simulink subsystem "Battery4Cell_SW_Res"  (R2022b)
settings: Solver=VariableStepAuto  StartTime=0.0  StopTime=10.0  RelTol=1e-3
model mask{V0=3.7, Ah=5.20, SOC1=70, SOC2=50, SOC3=60, SOC4=85, R=1}
  mask prompts: V0 "Nominal Voltage (V)"; Ah "Rated Capacity (Ah)"; SOC1 "Init SOC1 (%)"; SOC2 "Init SOC2 (%)"; SOC3 "Init SOC3 (%)"; SOC4 "Init SOC4 (%)"; R "Shunting Resistance"
undefined symbols (not defined in the file): Ion, Lithium
libraries: spsBatteryLib x4, spsIdealSwitchLib x4, spsParallelRLCBranchLib x4
settings Model: Creator=MAAM  LastModifiedBy=MAAM

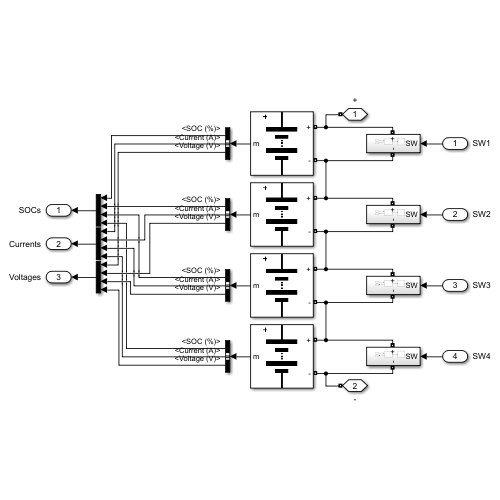
[thumbnail: Simulink's stored preview of the top-level diagram]
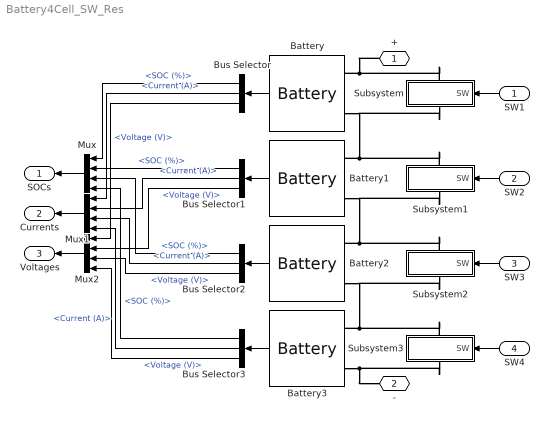
== system Battery4Cell_SW_Res ==
  SW1 : Inport
  SW2 : Inport  Port=2
  SW3 : Inport  Port=3
  SW4 : Inport  Port=4
  Battery : spsBatteryLib/Battery  BatType=Lithium-Ion  ShowTempParam=off  ThermalPreset=no  ShowAgeParam=off  NomV=V0  NomQ=Ah  SOC=SOC1  Batt_Tr=30  PresetModel=on  MaxQ=5.2  MinV=2.775  FullV=4.3068  Dis_rate=2.2609  R=0.0071154  Normal_OP=4.7026  expZone="[3.9974     0.25548]"  current=[6.5 13 32.5]  Units=Time  Tci=20  NomT=20  T2=-30  MaxQ2=4.8  FullV2=7.1  Normal_OP2=5.655  expZone2="[6.58           1]"  Rca=0.6  ti=2000  Dp=0  Neq0=0  Tsim=1e6  Ta1=25  Qeol=5.4*0.9  Reol=0.013333*1.2  Char_age=[2.3478, 3]  Dis_age=[2.3478, 10]  N1=1500  N2=10500  N3=1000  N4=1400  Ta2=45  N5=950
  Battery1 : spsBatteryLib/Battery  BatType=Lithium-Ion  ShowTempParam=off  ThermalPreset=no  ShowAgeParam=off  NomV=V0  NomQ=Ah  SOC=SOC2  Batt_Tr=30  PresetModel=on  MaxQ=5.2  MinV=2.775  FullV=4.3068  Dis_rate=2.2609  R=0.0071154  Normal_OP=4.7026  expZone="[3.9974     0.25548]"  current=[6.5 13 32.5]  Units=Time  Tci=20  NomT=20  T2=-30  MaxQ2=4.8  FullV2=7.1  Normal_OP2=5.655  expZone2="[6.58           1]"  Rca=0.6  ti=2000  Dp=0  Neq0=0  Tsim=1e6  Ta1=25  Qeol=5.4*0.9  Reol=0.013333*1.2  Char_age=[2.3478, 3]  Dis_age=[2.3478, 10]  N1=1500  N2=10500  N3=1000  N4=1400  Ta2=45  N5=950
  Battery2 : spsBatteryLib/Battery  BatType=Lithium-Ion  ShowTempParam=off  ThermalPreset=no  ShowAgeParam=off  NomV=V0  NomQ=Ah  SOC=SOC3  Batt_Tr=30  PresetModel=on  MaxQ=5.2  MinV=2.775  FullV=4.3068  Dis_rate=2.2609  R=0.0071154  Normal_OP=4.7026  expZone="[3.9974     0.25548]"  current=[6.5 13 32.5]  Units=Time  Tci=20  NomT=20  T2=-30  MaxQ2=4.8  FullV2=7.1  Normal_OP2=5.655  expZone2="[6.58           1]"  Rca=0.6  ti=2000  Dp=0  Neq0=0  Tsim=1e6  Ta1=25  Qeol=5.4*0.9  Reol=0.013333*1.2  Char_age=[2.3478, 3]  Dis_age=[2.3478, 10]  N1=1500  N2=10500  N3=1000  N4=1400  Ta2=45  N5=950
  Battery3 : spsBatteryLib/Battery  BatType=Lithium-Ion  ShowTempParam=off  ThermalPreset=no  ShowAgeParam=off  NomV=V0  NomQ=Ah  SOC=SOC4  Batt_Tr=30  PresetModel=on  MaxQ=5.2  MinV=2.775  FullV=4.3068  Dis_rate=2.2609  R=0.0071154  Normal_OP=4.7026  expZone="[3.9974     0.25548]"  current=[6.5 13 32.5]  Units=Time  Tci=20  NomT=20  T2=-30  MaxQ2=4.8  FullV2=7.1  Normal_OP2=5.655  expZone2="[6.58           1]"  Rca=0.6  ti=2000  Dp=0  Neq0=0  Tsim=1e6  Ta1=25  Qeol=5.4*0.9  Reol=0.013333*1.2  Char_age=[2.3478, 3]  Dis_age=[2.3478, 10]  N1=1500  N2=10500  N3=1000  N4=1400  Ta2=45  N5=950
  Bus Selector{,1..3} (4 alike) : BusSelector  OutputSignals=SOC (%),Current (A),Voltage (V)
  Mux : Mux
  Mux1 : Mux
  Mux2 : Mux
  Subsystem : Subsystem
      settings: PortSchema="{\"entries\":[{\"content\":{\"sides\":[{\"content\":{\"connectorIds\":[\"LConn1\"]},\"type\":\"ConnectorPlacement.EquallySpacedRectSide\",\"uuid\":\"eb8fffcd-a71c-4890-8fe1-844de9bb7049\"},{\"content\":{\"connectorIds\":[\"RConn1\"],\"side\":\"RIGHT\"},\"type\":\"ConnectorPlacement.EquallySpacedRectSide\",\"uuid\":\"5d4b0459-fb12-4785-8c10-98c9b0dba58c\"},{\"content\":{\"connectorIds\":[\"In1\"],\"side\":\"TOP\"},\"type\":\"ConnectorPlacement.EquallySpacedRectSide\",\"uuid\":\"54a7a206-2e51-43a0-a96b-a7248b1ad494\"}]},\"type\":\"ConnectorPlacement.EquallySpacedConnector\",\"uuid\":\"ba80d02d-3106-485f-afc0-f5d68efbd5a7\"}],\"packageUris\":[\"http://schema.mathworks.com/mf0/Connector/R2020b\"],\"version\":\"1.0\"}"
  Subsystem1 : Subsystem
      settings: PortSchema="{\"entries\":[{\"content\":{\"sides\":[{\"content\":{\"connectorIds\":[\"LConn1\"]},\"type\":\"ConnectorPlacement.EquallySpacedRectSide\",\"uuid\":\"eb8fffcd-a71c-4890-8fe1-844de9bb7049\"},{\"content\":{\"connectorIds\":[\"RConn1\"],\"side\":\"RIGHT\"},\"type\":\"ConnectorPlacement.EquallySpacedRectSide\",\"uuid\":\"5d4b0459-fb12-4785-8c10-98c9b0dba58c\"},{\"content\":{\"connectorIds\":[\"In1\"],\"side\":\"TOP\"},\"type\":\"ConnectorPlacement.EquallySpacedRectSide\",\"uuid\":\"54a7a206-2e51-43a0-a96b-a7248b1ad494\"}]},\"type\":\"ConnectorPlacement.EquallySpacedConnector\",\"uuid\":\"ba80d02d-3106-485f-afc0-f5d68efbd5a7\"}],\"packageUris\":[\"http://schema.mathworks.com/mf0/Connector/R2020b\"],\"version\":\"1.0\"}"
  Subsystem2 : Subsystem
      settings: PortSchema="{\"entries\":[{\"content\":{\"sides\":[{\"content\":{\"connectorIds\":[\"LConn1\"]},\"type\":\"ConnectorPlacement.EquallySpacedRectSide\",\"uuid\":\"eb8fffcd-a71c-4890-8fe1-844de9bb7049\"},{\"content\":{\"connectorIds\":[\"RConn1\"],\"side\":\"RIGHT\"},\"type\":\"ConnectorPlacement.EquallySpacedRectSide\",\"uuid\":\"5d4b0459-fb12-4785-8c10-98c9b0dba58c\"},{\"content\":{\"connectorIds\":[\"In1\"],\"side\":\"TOP\"},\"type\":\"ConnectorPlacement.EquallySpacedRectSide\",\"uuid\":\"54a7a206-2e51-43a0-a96b-a7248b1ad494\"}]},\"type\":\"ConnectorPlacement.EquallySpacedConnector\",\"uuid\":\"ba80d02d-3106-485f-afc0-f5d68efbd5a7\"}],\"packageUris\":[\"http://schema.mathworks.com/mf0/Connector/R2020b\"],\"version\":\"1.0\"}"
  Subsystem3 : Subsystem
      settings: PortSchema="{\"entries\":[{\"content\":{\"sides\":[{\"content\":{\"connectorIds\":[\"LConn1\"]},\"type\":\"ConnectorPlacement.EquallySpacedRectSide\",\"uuid\":\"eb8fffcd-a71c-4890-8fe1-844de9bb7049\"},{\"content\":{\"connectorIds\":[\"RConn1\"],\"side\":\"RIGHT\"},\"type\":\"ConnectorPlacement.EquallySpacedRectSide\",\"uuid\":\"5d4b0459-fb12-4785-8c10-98c9b0dba58c\"},{\"content\":{\"connectorIds\":[\"In1\"],\"side\":\"TOP\"},\"type\":\"ConnectorPlacement.EquallySpacedRectSide\",\"uuid\":\"54a7a206-2e51-43a0-a96b-a7248b1ad494\"}]},\"type\":\"ConnectorPlacement.EquallySpacedConnector\",\"uuid\":\"ba80d02d-3106-485f-afc0-f5d68efbd5a7\"}],\"packageUris\":[\"http://schema.mathworks.com/mf0/Connector/R2020b\"],\"version\":\"1.0\"}"
  + : PMIOPort  Side=Right
  - : PMIOPort  Port=2  Side=Right
  SOCs : Outport
  Currents : Outport  Port=2
  Voltages : Outport  Port=3
  wires:
  Mux2/1 -> Voltages/1
  Mux1/1 -> Currents/1
  Mux/1 -> SOCs/1
  Bus Selector1/3 -> Mux2/2  "<Voltage (V)>"
  Bus Selector2/3 -> Mux2/3  "<Voltage (V)>"
  Bus Selector3/3 -> Mux2/4  "<Voltage (V)>"
  Bus Selector3/2 -> Mux1/4  "<Current (A)>"
  Bus Selector2/2 -> Mux1/3  "<Current (A)>"
  Bus Selector/3 -> Mux2/1  "<Voltage (V)>"
  Bus Selector1/2 -> Mux1/2  "<Current (A)>"
  Bus Selector/2 -> Mux1/1  "<Current (A)>"
  Bus Selector/1 -> Mux/1  "<SOC (%)>"
  Bus Selector1/1 -> Mux/2  "<SOC (%)>"
  Bus Selector2/1 -> Mux/3  "<SOC (%)>"
  Bus Selector3/1 -> Mux/4  "<SOC (%)>"
  Battery2/1 -> Bus Selector2/1
  Battery3/1 -> Bus Selector3/1
  Battery1/1 -> Bus Selector1/1
  Battery/1 -> Bus Selector/1
  SW1/1 -> Subsystem/1(SW)
  SW2/1 -> Subsystem1/1(SW)
  SW3/1 -> Subsystem2/1(SW)
  SW4/1 -> Subsystem3/1(SW)
  connections:
  Subsystem1/LConn1 -- Subsystem/RConn1 -- Battery/LConn2 -- Battery1/LConn1
  Subsystem2/LConn1 -- Subsystem1/RConn1 -- Battery1/LConn2 -- Battery2/LConn1
  Subsystem3/LConn1 -- Subsystem2/RConn1 -- Battery2/LConn2 -- Battery3/LConn1
  Subsystem/LConn1 -- Battery/LConn1 -- +/RConn1
  Battery3/LConn2 -- Subsystem3/RConn1 -- -/RConn1

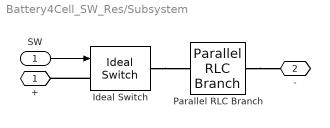
== system Battery4Cell_SW_Res/Subsystem ==
  SW : Inport
  Ideal Switch : spsIdealSwitchLib/Ideal Switch  Ron=0.001  Lon=0  IC=0  Rs=1e5  Cs=inf  Measurements=off
  Parallel RLC Branch : spsParallelRLCBranchLib/Parallel RLC Branch  LConnTagsString=a  RConnTagsString=__new0  BranchType=R  Resistance=R  Inductance=1e-3  SetiL0=off  InitialCurrent=0  Capacitance=1e-6  Setx0=off  InitialVoltage=0  Measurements=None
  + : PMIOPort  Side=Left
  - : PMIOPort  Port=2  Side=Right
  wires:
  SW/1 -> Ideal Switch/1
  connections:
  Ideal Switch/LConn1 -- +/RConn1
  Ideal Switch/RConn1 -- Parallel RLC Branch/LConn1
  Parallel RLC Branch/RConn1 -- -/RConn1

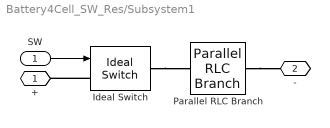
== system Battery4Cell_SW_Res/Subsystem1 ==
  SW : Inport
  Ideal Switch : spsIdealSwitchLib/Ideal Switch  Ron=0.001  Lon=0  IC=0  Rs=1e5  Cs=inf  Measurements=off
  Parallel RLC Branch : spsParallelRLCBranchLib/Parallel RLC Branch  LConnTagsString=a  RConnTagsString=__new0  BranchType=R  Resistance=R  Inductance=1e-3  SetiL0=off  InitialCurrent=0  Capacitance=1e-6  Setx0=off  InitialVoltage=0  Measurements=None
  + : PMIOPort  Side=Left
  - : PMIOPort  Port=2  Side=Right
  wires:
  SW/1 -> Ideal Switch/1
  connections:
  Parallel RLC Branch/RConn1 -- -/RConn1
  Ideal Switch/RConn1 -- Parallel RLC Branch/LConn1
  Ideal Switch/LConn1 -- +/RConn1

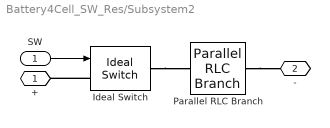
== system Battery4Cell_SW_Res/Subsystem2 ==
  SW : Inport
  Ideal Switch : spsIdealSwitchLib/Ideal Switch  Ron=0.001  Lon=0  IC=0  Rs=1e5  Cs=inf  Measurements=off
  Parallel RLC Branch : spsParallelRLCBranchLib/Parallel RLC Branch  LConnTagsString=a  RConnTagsString=__new0  BranchType=R  Resistance=R  Inductance=1e-3  SetiL0=off  InitialCurrent=0  Capacitance=1e-6  Setx0=off  InitialVoltage=0  Measurements=None
  + : PMIOPort  Side=Left
  - : PMIOPort  Port=2  Side=Right
  wires:
  SW/1 -> Ideal Switch/1
  connections:
  Ideal Switch/LConn1 -- +/RConn1
  Ideal Switch/RConn1 -- Parallel RLC Branch/LConn1
  Parallel RLC Branch/RConn1 -- -/RConn1

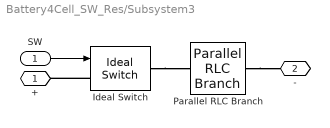
== system Battery4Cell_SW_Res/Subsystem3 ==
  SW : Inport
  Ideal Switch : spsIdealSwitchLib/Ideal Switch  Ron=0.001  Lon=0  IC=0  Rs=1e5  Cs=inf  Measurements=off
  Parallel RLC Branch : spsParallelRLCBranchLib/Parallel RLC Branch  LConnTagsString=a  RConnTagsString=__new0  BranchType=R  Resistance=R  Inductance=1e-3  SetiL0=off  InitialCurrent=0  Capacitance=1e-6  Setx0=off  InitialVoltage=0  Measurements=None
  + : PMIOPort  Side=Left
  - : PMIOPort  Port=2  Side=Right
  wires:
  SW/1 -> Ideal Switch/1
  connections:
  Parallel RLC Branch/RConn1 -- -/RConn1
  Ideal Switch/RConn1 -- Parallel RLC Branch/LConn1
  Ideal Switch/LConn1 -- +/RConn1
